simulink library "basic_EB"  (R2018b)
settings: Solver=ode45  StartTime=0.0  StopTime=10.0  RelTol=1e-3  EnableMultiTasking=on
settings Model: Creator=lena.frank  LastModifiedBy=P41573
settings DataIOCC: LimitDataPoints=on  SaveFormat=Array  SignalLoggingSaveFormat=ModelDataLogs
settings OptimizationCC: ExpressionDepthLimit=2147483647  LifeSpan=inf
settings DebuggingCC: UnderspecifiedInitializationDetection=Classic  MergeDetectMultiDrivingBlocksExec=none  SolverPrmCheckMsg=warning  FcnCallInpInsideContextMsg=warning  StateNameClashWarn=warning  SFUnexpectedBacktrackingDiag=warning  SFNoUnconditionalDefaultTransitionDiag=warning  SFExecutionAtInitializationDiag=none
settings HardwareCC: ProdBitPerPointer=32  ProdBitPerSizeT=32  ProdBitPerPtrDiffT=32  ProdLargestAtomicFloat=None  ProdIntDivRoundTo=Undefined  ProdEndianess=Unspecified  ProdWordSize=32  ProdHWDeviceType=32-bit Generic
settings ModelReferenceCC: PropagateSignalLabelsOutOfModel=off
settings SFSimCC: SimUseLocalCustomCode=off
settings RTWCC: RTWUseLocalCustomCode=off
settings CodeAppCC: StateflowObjectComments=on
settings GRTTargetCC: TargetLangStandard=C89/C90 (ANSI)  GeneratePreprocessorConditionals=Disable all  CombineOutputUpdateFcns=off  GRTInterface=on
settings ConfigComp: CovMetricSettings=dw  CovHtmlReporting=on  CovSaveCumulativeToWorkspaceVar=on  CovSaveSingleToWorkspaceVar=on  CovExternalEMLEnable=off

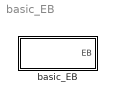
== system basic_EB ==
  basic_EB : Subsystem  InitFcn=load('EB.mat')  mask(basic_EB){eID=Power only, f=50, v1=230, p1=0, pf1=1, v2=230, p2=0, pf2=1, v3=230, p3=0, pf3=1}
      mask prompts: eID "ID for electric calculation"; f "frequency [Hz]"; v1 "voltage to ground [V]"; p1 "active  power [VA]"; pf1 "power factor[-]"; v2 "voltage to ground [V]"; p2 "active  power [VA]"; pf2 "power factor[-]"; v3 "voltage to ground [V]"; p3 "active  power [VA]"; pf3 "power factor[-]"
      mask help: Create a constant Electric Bus.
      mask Help: web(fullfile(path_carnot('help'),'basic_EB.html'),'-helpbrowser')
      mask TypeOptions eID: ID/eID
      mask TypeOptions f: f/Value
      mask TypeOptions v1: v1/Value
      mask TypeOptions p1: p1/Value
      mask TypeOptions pf1: pf1/Value
      mask TypeOptions v2: v2/Value
      mask TypeOptions p2: p2/Value
      mask TypeOptions pf2: pf2/Value
      mask TypeOptions v3: v3/Value
      mask TypeOptions p3: p3/Value
      mask TypeOptions pf3: pf3/Value
      mask DialogControl ParameterTabVar03 Prompt: Common
      mask DialogControl ParameterTabVar0 Prompt: Line 1
      mask DialogControl ParameterTabVar01 Prompt: Line2
      mask DialogControl ParameterTabVar02 Prompt: Line3

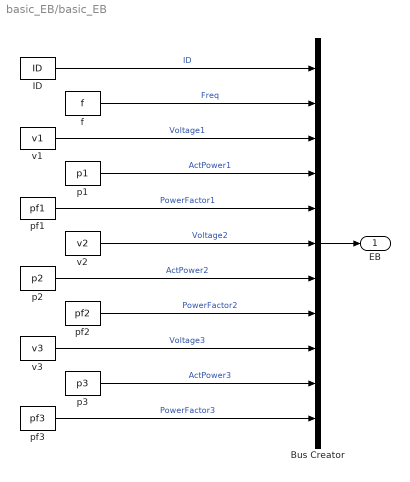
== system basic_EB/basic_EB ==
  Bus Creator : BusCreator  InitFcn=load THB.mat  Inputs=11  OutDataTypeStr=Bus: EB
      settings: InheritFromInputs=off
  ID : Constant  Value=ID  mask{eID=Power only}
      mask prompts: eID "ID for electric calculation"
      mask init:
      | ID = eID;
      mask TypeOptions eID: Power only | DC | AC_1P | AC_3P
  f : Constant  Value=f
  p1 : Constant  Value=p1
  p2 : Constant  Value=p2
  p3 : Constant  Value=p3
  pf1 : Constant  Value=pf1
  pf2 : Constant  Value=pf2
  pf3 : Constant  Value=pf3
  v1 : Constant  Value=v1
  v2 : Constant  Value=v2
  v3 : Constant  Value=v3
  EB : Outport
  wires:
  v2/1 -> Bus Creator/6  "Voltage2"
  f/1 -> Bus Creator/2  "Freq"
  pf1/1 -> Bus Creator/5  "PowerFactor1"
  p1/1 -> Bus Creator/4  "ActPower1"
  v1/1 -> Bus Creator/3  "Voltage1"
  ID/1 -> Bus Creator/1  "ID"
  Bus Creator/1 -> EB/1
  p3/1 -> Bus Creator/10  "ActPower3"
  v3/1 -> Bus Creator/9  "Voltage3"
  pf3/1 -> Bus Creator/11  "PowerFactor3"
  p2/1 -> Bus Creator/7  "ActPower2"
  pf2/1 -> Bus Creator/8  "PowerFactor2"
